simulink model "failed_string_test"  (R2019a)
settings: Solver=VariableStepAuto  StartTime=0.0  StopTime=10.0  RelTol=1e-3
settings Model: Creator=marco  LastModifiedBy=marco

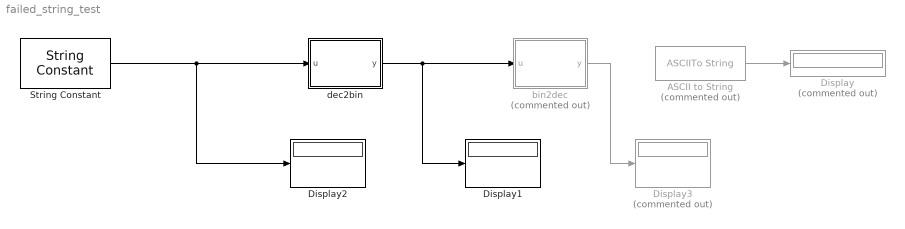
== system failed_string_test ==
  ASCII to String : ASCIIToString  Commented=on
  Display : Display  Commented=on
  Display1 : Display
  Display2 : Display
  Display3 : Display  Commented=on
  String Constant : StringConstant  String="\"ab\""
  bin2dec : MATLAB Function  Commented=on  TreatAsAtomicUnit=on
  "dec2bin " : MATLAB Function  TreatAsAtomicUnit=on
  wires:
  String Constant/1 -> "dec2bin "/1(u), Display2/1
  ASCII to String/1 -> Display/1
  bin2dec/1(y) -> Display3/1
  "dec2bin "/1(y) -> Display1/1, bin2dec/1(u)

== matlab function failed_string_test/bin2dec ==
  data: y output [..100]; u input [..100]
function y = fcn(u)

y = bin2dec(char(u));

== matlab function failed_string_test/dec2bin  ==
  data: u input size=1; y output size=100 [0..100]
function y = fcn(u)

y = dec2bin(u);
